simulink model "MySimModel"  (R2024b)
settings: Solver=VariableStepAuto  StartTime=0.0  StopTime=10.0  RelTol=1e-3
settings Model: Creator=xinxing  LastModifiedBy=xinxing

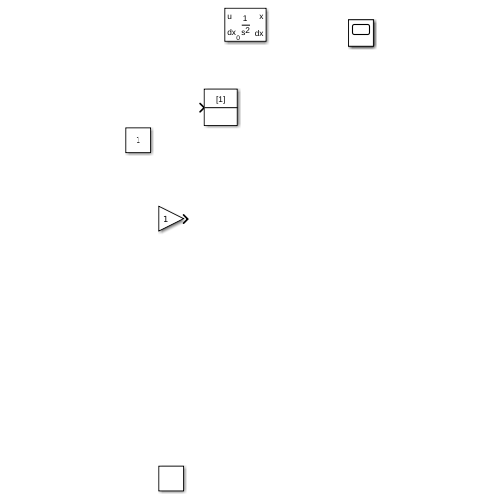
[thumbnail: Simulink's stored preview of the top-level diagram]
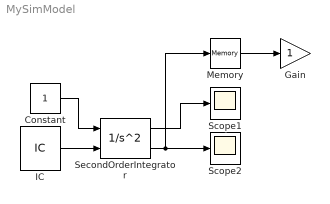
== system MySimModel ==
  Constant : Constant
  Gain : Gain
  IC : InitialCondition
  Memory : Memory
  Scope1 : Scope
  Scope2 : Scope
  SecondOrderIntegrator : SecondOrderIntegrator  ICSourceDXDT=external
  wires:
  Memory/1 -> Gain/1
  SecondOrderIntegrator/2 -> Memory/1, Scope2/1
  SecondOrderIntegrator/1 -> Scope1/1
  IC/1 -> SecondOrderIntegrator/2
  Constant/1 -> SecondOrderIntegrator/1
